simulink model "battery_ecm"  (R2026a)
settings: Solver=VariableStepAuto  StopTime=3591.234
undefined symbols (not defined in the file): OCV_table, SOC_table
settings Model: Creator=rohith  LastModifiedBy=rohith

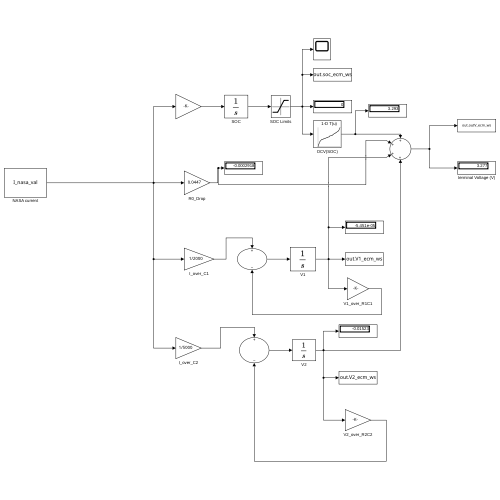
[thumbnail: Simulink's stored preview of the top-level diagram]
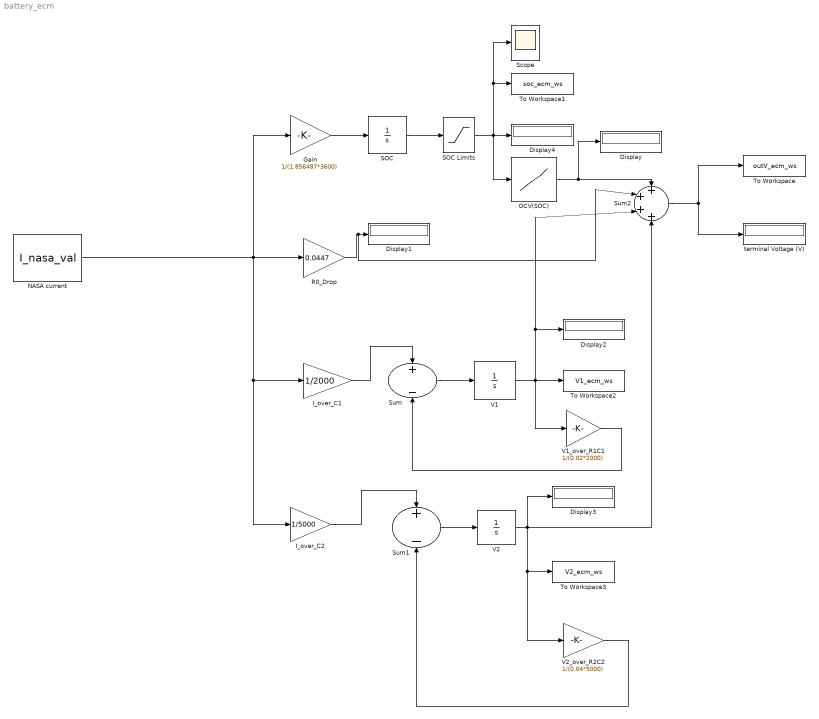
== system battery_ecm ==
  Display{,1..4} (5 alike) : Display
  Gain : Gain  Gain=1/(1.856487*3600)
  I_over_C1 : Gain  Gain=1/2000
  I_over_C2 : Gain  Gain=1/5000
  NASA current : FromWorkspace  VariableName=I_nasa_val
  OCV(SOC) : Lookup_n-D  NumberOfTableDimensions=1  BreakpointsForDimension1=SOC_table  Table=OCV_table  InternalRulePriority=Speed  RndMeth=Simplest
  R0_Drop : Gain  Gain=0.0447
  SOC : Integrator  InitialCondition=1
  SOC Limits : Saturate  UpperLimit=1  LowerLimit=0
  Scope : Scope
      settings: ActiveDisplayYMinimum=-1  ActiveDisplayYMaximum=1
  Sum : Sum  Inputs=+-
  Sum1 : Sum  Inputs=+-
  Sum2 : Sum  Inputs=++++
  To Workspace : ToWorkspace  VariableName=outV_ecm_ws  SaveFormat=Timeseries  SampleTime=-1
  To Workspace1 : ToWorkspace  VariableName=soc_ecm_ws  SaveFormat=Timeseries  SampleTime=-1
  To Workspace2 : ToWorkspace  VariableName=V1_ecm_ws  SaveFormat=Timeseries  SampleTime=-1
  To Workspace3 : ToWorkspace  VariableName=V2_ecm_ws  SaveFormat=Timeseries  SampleTime=-1
  V1 : Integrator
  V1_over_R1C1 : Gain  Gain=1/(0.02*2000)
  V2 : Integrator
  V2_over_R2C2 : Gain  Gain=1/(0.04*5000)
  terminal Voltage (V) : Display
  wires:
  Gain/1 -> SOC/1
  SOC/1 -> SOC Limits/1
  SOC Limits/1 -> To Workspace1/1, Scope/1, Display4/1, OCV(SOC)/1
  OCV(SOC)/1 -> Sum2/1, Display/1
  R0_Drop/1 -> Sum2/2, Display1/1
  I_over_C1/1 -> Sum/1
  Sum/1 -> V1/1
  V1/1 -> To Workspace2/1, V1_over_R1C1/1, Sum2/3, Display2/1
  V1_over_R1C1/1 -> Sum/2
  I_over_C2/1 -> Sum1/1
  Sum1/1 -> V2/1
  V2/1 -> To Workspace3/1, V2_over_R2C2/1, Display3/1, Sum2/4
  V2_over_R2C2/1 -> Sum1/2
  Sum2/1 -> terminal Voltage (V)/1, To Workspace/1
  NASA current/1 -> I_over_C2/1, I_over_C1/1, Gain/1, R0_Drop/1
